simulink model "F4PhantomRunningModel2021a"  (R2021a)
settings: Solver=ode4  StartTime=0.0  StopTime=tf  FixedStep=Ts  RelTol=1e-3
model workspace (MAT data in the model file):
  PositionStateAttributes = {'Xe', 'Ye', 'Ze'}
  QuaternionStateAttributes = {'qr', 'qi', 'qj', 'qk'}
  RotationStateAttributes = {'p', 'q', 'r'}
  VelocityStateAttributes = {'U', 'v', 'w'}
values from neighbouring files (symbols this model uses):
  Hw3Coeffs = [c_L_alpha c_L_delta_E c_L_i_H c_m_alpha c_m_delta_E c_m_i_H c_L_alphadot c_L_q c_m_alphadot c_m_q c_D_alpha]    [F4ModelCode.m]    (also in F4ModelCodeV2.m; F4ModelCodeV2Q2PartD.m; F4PhantomModelCode.m = [c_L_alpha c_L_delta_E c_L_i_H c_m_alpha c_m_delta_E c_m_i_H)
  Hw4Coeffs = [c_Y_beta c_Y_delta_A c_Y_delta_R c_n_beta c_n_delta_A c_n_delta_R c_l_beta c_l_delta_A c_l_delta_R c_l_p c_Y_p c_n_p c_l_r c_Y_r c_n_r]    [F4ModelCode.m]    (also in F4ModelCodeV2.m; F4ModelCodeV2Q2PartD.m; F4PhantomModelCode.m)
  InitialInputs = [qbar1 S_ft2 c_D_1 c_L_1 cbar_ft c_m_1 uv b_ft alphadot]    [F4ModelCode.m]    (also in F4ModelCodeV2.m; F4ModelCodeV2Q2PartD.m)
  uCoeffs = [c_L_u c_D_u c_m_u]    [F4ModelCode.m]    (also in F4ModelCodeV2.m; F4ModelCodeV2Q2PartD.m; F4PhantomModelCode.m = [c_L_u c_D_u])
  uk = [c_D_delta_E c_D_q c_D_i_H c_Y_1 c_Y_betadot c_l_betadot c_n_1 c_n_betadot]    [F4ModelCode.m]    (also in F4ModelCodeV2.m; F4ModelCodeV2Q2PartD.m)
  V_P_1 = 875.6    [F4ModelCode.m]    (also in F4ModelCodeV2.m; F4ModelCodeV2Q2PartD.m; F4PhantomModelCode.m = 0)
libraries: shared6dof x1
settings Model: Creator=Owner  LastModifiedBy=billy
settings DataIOCC: ReturnWorkspaceOutputs=off
settings HardwareCC: ProdHWDeviceType=AMD->x86-64 (Windows64)
settings RTWCC: Description=Generic Real-Time Target  DLArmComputeVersion=20.02.1

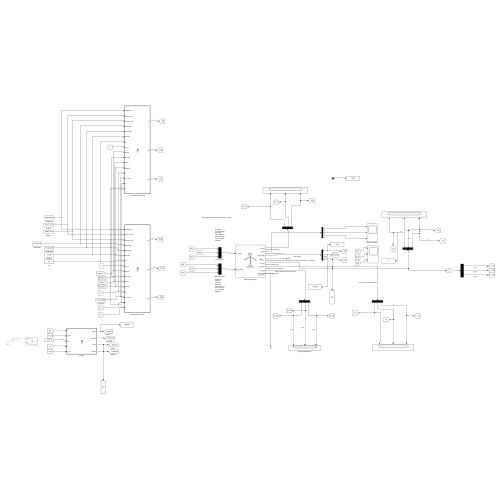
[thumbnail: Simulink's stored preview of the top-level diagram]
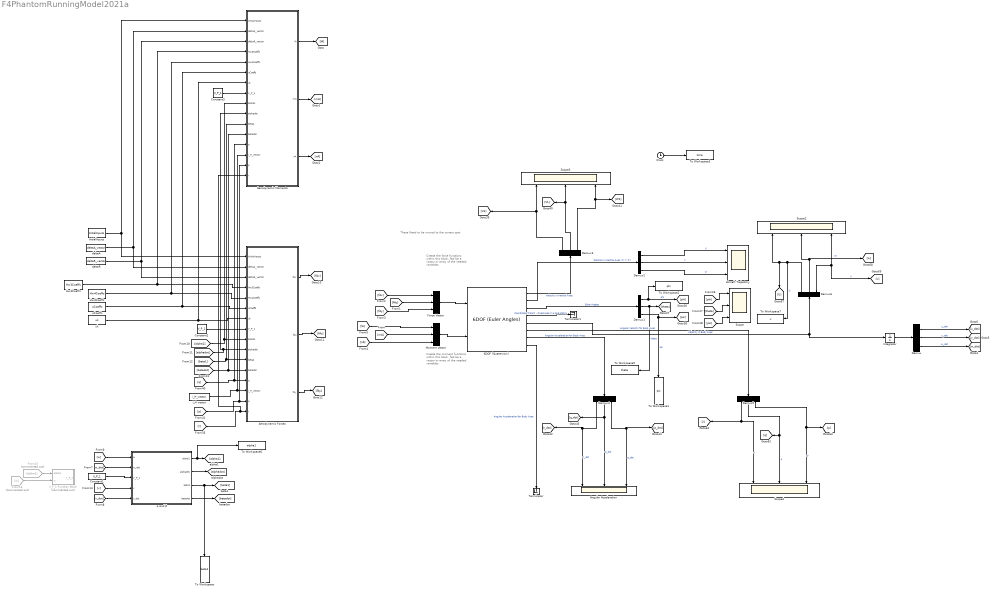
== system F4PhantomRunningModel2021a ==
  note: These Need to be moved to the correct spot
  note: Create the moment functions within this block, fed be a vector or array of the needed variables
  note: Create the force functions within this block, fed be a vector or array of the needed variables
  6DOF (Quaternion) : shared6dof/6DOF (Euler Angles)  units=English (Velocity in ft/s)  mtype=Fixed  rep=Quaternion  xme_0=InitialInertialPosition  Vm_0=InitialVelocity  eul_0=InitialEulerOrientation  pm_0=InitialRotationRates  mass_0=mass  mass_e=0.5  mass_f=2.0  inertia=I  inertia_e=eye(3)  inertia_f=2*eye(3)  k_quat=1.0  vre_flag=on  abi_flag=off  aMode=0  xme_statename=PositionStateAttributes  Vm_statename=VelocityStateAttributes  eul_statename=''  quat_statename=QuaternionStateAttributes  pm_statename=RotationStateAttributes  mass_statename=''
  Aerodynamic Forces : MATLAB Function  TreatAsAtomicUnit=on
  Aerodynamic Moments : MATLAB Function  TreatAsAtomicUnit=on
  Aircraft Trajectory : Scope  NumInputPorts=3
  Angular Acceleration : Scope  NumInputPorts=3
  Clock : Clock
  Constant1 : Constant  Value=V_P_1
  Constant2 : Constant  Value=V_P_1
  Constant3 : Constant  Value=V_P_1
  Demux{,1..6} (7 alike) : Demux  Outputs=3
  Force Vector : Mux  Inputs=3
  From15 : From  Commented=on  GotoTag=alpha1
  From16 : From  Commented=on  GotoTag=w
  Hw3Coeffs : Constant  Value=Hw3Coeffs
  Hw4Coeffs : Constant  Value=Hw4Coeffs
  InitialInputs : Constant  Value=InitialInputs
  Integrator : Integrator
  Moment Vector : Mux  Inputs=3
  Scope{,2..4} (4 alike) : Scope  NumInputPorts=3
  Terminator : Terminator
  Terminator1 : Terminator
  To Workspace : ToWorkspace  VariableName=beta1  SampleTime=-1
      settings: Save2DSignal=2-D array (concatenate along first dimension)
  To Workspace1 : ToWorkspace  VariableName=psi  SampleTime=-1
      settings: Save2DSignal=2-D array (concatenate along first dimension)
  To Workspace2 : ToWorkspace  VariableName=phi  SampleTime=-1
      settings: Save2DSignal=2-D array (concatenate along first dimension)
  To Workspace3 : ToWorkspace  VariableName=time  SaveFormat=Timeseries  SampleTime=-1
  To Workspace5 : ToWorkspace  VariableName=theta  SampleTime=-1
      settings: Save2DSignal=2-D array (concatenate along first dimension)
  To Workspace6 : ToWorkspace  VariableName=alpha1  SampleTime=-1
      settings: Save2DSignal=2-D array (concatenate along first dimension)
  To Workspace7 : ToWorkspace  VariableName=u  SampleTime=-1
      settings: Save2DSignal=2-D array (concatenate along first dimension)
  V_P_1 Function Block : MATLAB Function  Commented=on  TreatAsAtomicUnit=on
  "deltaA " : FromWorkspace  VariableName=deltaA_vector  OutDataTypeStr=double
  "deltaR " : FromWorkspace  VariableName=deltaR_vector  OutDataTypeStr=double
  "i_H vector " : FromWorkspace  VariableName=i_H_vector
  uCoeffs : Constant  Value=uCoeffs
  uk : Constant  Value=uk
  α and β : MATLAB Function  TreatAsAtomicUnit=on
  wires:
  Force Vector/1 -> 6DOF (Quaternion)/1
  6DOF (Quaternion)/1 -> Demux3/1  "Velocity in Inertial Axes"
  6DOF (Quaternion)/2 -> Demux2/1  "Position in Inertial Axes (X' Y' Z')"
  6DOF (Quaternion)/3 -> Demux1/1  "Euler Angles"
  6DOF (Quaternion)/4 -> Terminator1/1  "Coordinate Transformation from Flat Earth axes to Body-Fixed axes in a 3x3 Matrix"
  6DOF (Quaternion)/5 -> Integrator/1, Demux6/1  "Velocity in Body Axes"
  6DOF (Quaternion)/6 -> Demux5/1  "Angular Velocity for Body Axes"
  6DOF (Quaternion)/7 -> Demux4/1  "Angular Acceleration for Body Axes"
  6DOF (Quaternion)/8 -> Terminator/1  "Angular Acceleration for Body Axes"
  Aerodynamic Forces/1(fAx) -> [fAx]
  Aerodynamic Forces/2(fAz) -> [fAz]
  Aerodynamic Forces/3(fAy) -> [fAy]
  Moment Vector/1 -> 6DOF (Quaternion)/2
  [fAz] -> Force Vector/2
  [fAx] -> Force Vector/1
  [mA] -> Moment Vector/2
  [fAy] -> Force Vector/3
  [nA] -> Moment Vector/3
  [lA] -> Moment Vector/1
  Demux1/1 -> To Workspace2/1, [phi]  "phi"
  Demux1/2 -> To Workspace5/1, [theta]  "theta"
  Demux1/3 -> [psi], To Workspace1/1  "psi"
  [phi] -> Scope/1
  [theta] -> Scope/2
  [psi] -> Scope/3
  Demux2/1 -> Aircraft Trajectory/1  "X'"
  Demux2/2 -> Aircraft Trajectory/2  "Y'"
  Demux2/3 -> Aircraft Trajectory/3  "Z'"
  Demux3/1 -> Scope3/1, [U1]
  Demux3/2 -> [V1], Scope3/2
  Demux3/3 -> Scope3/3, [W1]
  Demux4/1 -> [r_dot], Angular Acceleration/1  "r_dot"
  Demux4/2 -> [q_dot], Angular Acceleration/2  "q_dot"
  Demux4/3 -> [p_dot], Angular Acceleration/3  "p_dot"
  Demux5/1 -> [r], Scope4/1  "r"
  Demux5/2 -> [q], Scope4/2  "q"
  Demux5/3 -> [p], Scope4/3  "p"
  [p] -> Aerodynamic Moments/15(p), Aerodynamic Forces/15(p)
  [r] -> Aerodynamic Moments/16(r), Aerodynamic Forces/16(r)
  α and β/1(alpha1) -> To Workspace6/1, [alpha1]
  α and β/4(betadot) -> [betadot]
  α and β/3(beta1) -> [beta1], To Workspace/1
  α and β/2(alphadot) -> [alphadot]
  Demux6/3 -> [v], Scope2/3  "V"
  Demux6/2 -> [w], Scope2/2  "W"
  Demux6/1 -> To Workspace7/1, Scope2/1, [U]  "U"
  [q] -> Aerodynamic Moments/13(q), Aerodynamic Forces/13(q)
  InitialInputs/1 -> Aerodynamic Moments/1(InitialInputs), Aerodynamic Forces/1(InitialInputs)
  "deltaA "/1 -> Aerodynamic Moments/2(deltaA_vector), Aerodynamic Forces/2(deltaA_vector)
  Hw3Coeffs/1 -> Aerodynamic Moments/4(Hw3Coeffs), Aerodynamic Forces/4(Hw3Coeffs)
  Hw4Coeffs/1 -> Aerodynamic Moments/5(Hw4Coeffs), Aerodynamic Forces/5(Hw4Coeffs)
  uCoeffs/1 -> Aerodynamic Moments/6(uCoeffs), Aerodynamic Forces/6(uCoeffs)
  uk/1 -> Aerodynamic Moments/7(uk), Aerodynamic Forces/7(uk)
  "i_H vector "/1 -> Aerodynamic Moments/14(i_H_vector), Aerodynamic Forces/14(i_H_vector)
  [alpha1] -> Aerodynamic Forces/9(alpha1), Aerodynamic Moments/9(alpha1)
  [alphadot] -> Aerodynamic Forces/10(alphadot), Aerodynamic Moments/10(alphadot)
  [beta1] -> Aerodynamic Forces/11(beta1), Aerodynamic Moments/11(beta1)
  [betadot] -> Aerodynamic Forces/12(betadot), Aerodynamic Moments/12(betadot)
  Integrator/1 -> Demux/1
  Demux/1 -> [u_dot]  "u_dot"
  Demux/2 -> [v_dot]  "v_dot"
  Demux/3 -> [w_dot]  "w_dot"
  [w_dot] -> α and β/2(w_dot)
  [v_dot] -> α and β/5(v_dot)
  [w] -> α and β/1(w)
  [v] -> α and β/4(v)
  From15/1 -> V_P_1 Function Block/1(alpha1)
  From16/1 -> V_P_1 Function Block/2(w)
  "deltaR "/1 -> Aerodynamic Moments/3(deltaR_vector), Aerodynamic Forces/3(deltaR_vector)
  Aerodynamic Moments/1(lA) -> [lA]
  Aerodynamic Moments/2(mA) -> [mA]
  Aerodynamic Moments/3(nA) -> [nA]
  Constant1/1 -> α and β/3(V_P_1)
  Constant2/1 -> Aerodynamic Forces/8(V_P_1)
  Constant3/1 -> Aerodynamic Moments/8(V_P_1)
  Clock/1 -> To Workspace3/1

== matlab function F4PhantomRunningModel2021a/Aerodynamic Forces ==
  data: InitialInputs input; deltaA_vector input; deltaR_vector input; Hw3Coeffs input; Hw4Coeffs input; uCoeffs input; uk input; V_P_1 input; alpha1 input; alphadot input; beta1 input; betadot input; q input; i_H_vector input; fAx output; fAz output; fAy output; p input; r input
function [ fAx, fAz,  fAy]  = fcn(InitialInputs, deltaA_vector, deltaR_vector, Hw3Coeffs, Hw4Coeffs, uCoeffs, uk, V_P_1, alpha1, alphadot, beta1, betadot, q, i_H_vector, p, r)
qbar1 = InitialInputs(1); S_ft2 = InitialInputs(2); c_D_1 = InitialInputs(3); c_L_1 = InitialInputs(4); cbar_ft = InitialInputs(5); c_m_1 = InitialInputs(6); uv = InitialInputs(7); b_ft = InitialInputs(8);
% deltaA_vector = CSv(1); deltaR_vector = CSv(2); deltaS_vector = CSv(3); 
% deltaA = CSc(1); deltaS = CSc(2); deltaR = CSc(3);
c_L_alpha = Hw3Coeffs(1); c_L_delta_E = Hw3Coeffs(2); c_L_i_H = Hw3Coeffs(3); c_m_alpha = Hw3Coeffs(4); c_m_delta_E = Hw3Coeffs(5); c_m_i_H = Hw3Coeffs(6); c_L_alphadot = Hw3Coeffs(7); c_L_q = Hw3Coeffs(8); c_m_alphadot = Hw3Coeffs(9); c_m_q = Hw3Coeffs(10); c_D_alpha = Hw3Coeffs(11);
c_Y_beta = Hw4Coeffs(1); c_Y_delta_A = Hw4Coeffs(2); c_Y_delta_R = Hw4Coeffs(3); c_n_beta = Hw4Coeffs(4); c_n_delta_A = Hw4Coeffs(5); c_n_delta_R = Hw4Coeffs(6); c_l_beta = Hw4Coeffs(7); c_l_delta_A = Hw4Coeffs(8); c_l_delta_R = Hw4Coeffs(9); c_l_p = Hw4Coeffs(10); c_Y_p = Hw4Coeffs(11); c_n_p = Hw4Coeffs(12); c_l_r = Hw4Coeffs(13); c_Y_r = Hw4Coeffs(14); c_n_r = Hw4Coeffs(15);
c_L_u = uCoeffs(1); c_D_u = uCoeffs(2); c_m_u = uCoeffs(3); 
c_D_delta_E = uk(1);  c_D_q = uk(2); c_D_i_H = uk(3); c_Y_1 = uk(4); c_Y_betadot = uk(5); c_l_betadot = uk(6); c_n_1 = uk(7); c_n_betadot = uk(8);

deltaE = 0;

%FAx = -qbar1*S_ft2*c_D_1;
fAx = (qbar1*S_ft2)*(((-(c_D_u+(2*c_D_1)))*(uv/V_P_1)) + ((c_D_alpha + c_L_1)*(alpha1)) - c_D_alpha*((alphadot*cbar_ft)/(2*V_P_1)) - c_D_q*((q*cbar_ft)/(2*V_P_1)) - (c_D_delta_E*deltaE)-(c_D_i_H*i_H_vector));

%FAz = -qbar1*S_ft2*c_L_1;
fAz = (qbar1*S_ft2)*(((-(c_L_u+(2*c_L_1)))*(uv/V_P_1)) + ((c_L_alpha + c_D_1)*(alpha1)) - c_L_alphadot*((alphadot*cbar_ft)/(2*V_P_1)) - c_L_q*((q*cbar_ft)/(2*V_P_1)) - (c_L_delta_E*deltaE)-(c_L_i_H*i_H_vector));

%FAy = -qbar1*S_ft2*c_Y_1;
fAy = -qbar1*S_ft2 * ((c_Y_beta*beta1) + c_Y_betadot * ((betadot*b_ft)/(2*V_P_1)) + c_Y_p*((p*b_ft)/(2*V_P_1)) + c_Y_r * ((r*b_ft)/(2*V_P_1)) +(c_Y_delta_A * deltaA_vector) + (c_Y_delta_R*deltaR_vector));

%LA = -qbar1*S_ft2*b_ft*c_L_1;
% lA = -qbar1*S_ft2*b_ft*((c_l_beta*beta1) + c_l_betadot * ((betadot*b_ft)/(2*V_P_1)) + c_l_p*((p*b_ft)/(2*V_P_1)) + c_l_r * ((r*b_ft)/(2*V_P_1)) +(c_l_delta_A * deltaA_vector) + (c_l_delta_R*deltaR_vector));
% 
% %MA = -qbar1*S_ft2*cbar_ft*c_m_1; %%%%This line is throwing an error
% mA = (qbar1*S_ft2*cbar_ft)*(((-(c_m_u+(2*c_m_1)))*(uv/V_P_1)) + (c_m_alpha*alpha1) + c_m_alphadot*((alphadot*cbar_ft)/(2*V_P_1)) + c_m_q*((q*cbar_ft)/(2*V_P_1)) + (c_m_delta_E*deltaE)+(c_L_i_H*i_H_vector));
% 
% %NA = -qbar1*S_ft2*b_ft*c_n_1;
% nA = -qbar1*S_ft2*b_ft*((c_n_beta*beta1) + c_n_betadot * ((betadot*b_ft)/(2*V_P_1)) + c_n_p*((p*b_ft)/(2*V_P_1)) + c_n_r * ((r*b_ft)/(2*V_P_1)) +(c_n_delta_A * deltaA_vector) + (c_n_delta_R*deltaR_vector));

%Need to get rid of fAy and lA and nA, leave MA and mA

== matlab function F4PhantomRunningModel2021a/α and β ==
  data: w input; alpha1 output; alphadot output; beta1 output; w_dot input; V_P_1 input; v input; v_dot input; betadot output
function [alpha1, alphadot, beta1, betadot] = fcn(w, w_dot, V_P_1, v, v_dot)

alpha1 = w/V_P_1;

alphadot = w_dot/V_P_1;

beta1 = v/V_P_1;

betadot = v_dot/V_P_1;

== matlab function F4PhantomRunningModel2021a/V_P_1 Function Block ==
  data: alpha1 input; V_P_1 output; w input
function V_P_1 = fcn(alpha1,w)

alpha1 = deg2rad(alpha1); 
V_P_1 = w/alpha1;

== matlab function F4PhantomRunningModel2021a/Aerodynamic Moments ==
  data: InitialInputs input; deltaA_vector input; deltaR_vector input; Hw3Coeffs input; Hw4Coeffs input; uCoeffs input; uk input; V_P_1 input; alpha1 input; alphadot input; beta1 input; betadot input; q input; i_H_vector input; lA output; mA output; nA output; p input; r input
function [lA,  mA, nA]  = fcn(InitialInputs, deltaA_vector, deltaR_vector, Hw3Coeffs, Hw4Coeffs, uCoeffs, uk, V_P_1, alpha1, alphadot, beta1, betadot, q, i_H_vector, p, r)
qbar1 = InitialInputs(1); S_ft2 = InitialInputs(2); c_D_1 = InitialInputs(3); c_L_1 = InitialInputs(4); cbar_ft = InitialInputs(5); c_m_1 = InitialInputs(6); uv = InitialInputs(7); b_ft = InitialInputs(8);
% deltaA_vector = CSv(1); deltaR_vector = CSv(2); deltaS_vector = CSv(3); 
% deltaA = CSc(1); deltaS = CSc(2); deltaR = CSc(3);
c_L_alpha = Hw3Coeffs(1); c_L_delta_E = Hw3Coeffs(2); c_L_i_H = Hw3Coeffs(3); c_m_alpha = Hw3Coeffs(4); c_m_delta_E = Hw3Coeffs(5); c_m_i_H = Hw3Coeffs(6); c_L_alphadot = Hw3Coeffs(7); c_L_q = Hw3Coeffs(8); c_m_alphadot = Hw3Coeffs(9); c_m_q = Hw3Coeffs(10); c_D_alpha = Hw3Coeffs(11);
c_Y_beta = Hw4Coeffs(1); c_Y_delta_A = Hw4Coeffs(2); c_Y_delta_R = Hw4Coeffs(3); c_n_beta = Hw4Coeffs(4); c_n_delta_A = Hw4Coeffs(5); c_n_delta_R = Hw4Coeffs(6); c_l_beta = Hw4Coeffs(7); c_l_delta_A = Hw4Coeffs(8); c_l_delta_R = Hw4Coeffs(9); c_l_p = Hw4Coeffs(10); c_Y_p = Hw4Coeffs(11); c_n_p = Hw4Coeffs(12); c_l_r = Hw4Coeffs(13); c_Y_r = Hw4Coeffs(14); c_n_r = Hw4Coeffs(15);
c_L_u = uCoeffs(1); c_D_u = uCoeffs(2); c_m_u = uCoeffs(3); 
c_D_delta_E = uk(1);  c_D_q = uk(2); c_D_i_H = uk(3); c_Y_1 = uk(4); c_Y_betadot = uk(5); c_l_betadot = uk(6); c_n_1 = uk(7); c_n_betadot = uk(8);

deltaE = 0;

% %FAx = -qbar1*S_ft2*c_D_1;
% fAx = (qbar1*S_ft2)*(((-(c_D_u+(2*c_D_1)))*(uv/V_P_1)) + ((c_D_alpha + c_L_1)*(alpha1)) - c_D_alpha*((alphadot*cbar_ft)/(2*V_P_1)) - c_D_q*((q*cbar_ft)/(2*V_P_1)) - (c_D_delta_E*deltaE)-(c_D_i_H*i_H_vector));
% 
% %FAz = -qbar1*S_ft2*c_L_1;
% fAz = (qbar1*S_ft2)*(((-(c_L_u+(2*c_L_1)))*(uv/V_P_1)) + ((c_L_alpha + c_D_1)*(alpha1)) - c_L_alphadot*((alphadot*cbar_ft)/(2*V_P_1)) - c_L_q*((q*cbar_ft)/(2*V_P_1)) - (c_L_delta_E*deltaE)-(c_L_i_H*i_H_vector));
% 
% %FAy = -qbar1*S_ft2*c_Y_1;
% fAy = -qbar1*S_ft2 * ((c_Y_beta*beta1) + c_Y_betadot * ((betadot*b_ft)/(2*V_P_1)) + c_Y_p*((p*b_ft)/(2*V_P_1)) + c_Y_r * ((r*b_ft)/(2*V_P_1)) +(c_Y_delta_A * deltaA_vector) + (c_Y_delta_R*deltaR_vector));

%LA = -qbar1*S_ft2*b_ft*c_L_1;
lA = -qbar1*S_ft2*b_ft*((c_l_beta*beta1) + c_l_betadot * ((betadot*b_ft)/(2*V_P_1)) + c_l_p*((p*b_ft)/(2*V_P_1)) + c_l_r * ((r*b_ft)/(2*V_P_1)) +(c_l_delta_A * deltaA_vector) + (c_l_delta_R*deltaR_vector));
% 
% %MA = -qbar1*S_ft2*cbar_ft*c_m_1; %%%%This line is throwing an error
mA = (qbar1*S_ft2*cbar_ft)*(((-(c_m_u+(2*c_m_1)))*(uv/V_P_1)) + (c_m_alpha*alpha1) + c_m_alphadot*((alphadot*cbar_ft)/(2*V_P_1)) + c_m_q*((q*cbar_ft)/(2*V_P_1)) + (c_m_delta_E*deltaE)+(c_L_i_H*i_H_vector));
% 
% %NA = -qbar1*S_ft2*b_ft*c_n_1;
nA = -qbar1*S_ft2*b_ft*((c_n_beta*beta1) + c_n_betadot * ((betadot*b_ft)/(2*V_P_1)) + c_n_p*((p*b_ft)/(2*V_P_1)) + c_n_r * ((r*b_ft)/(2*V_P_1)) +(c_n_delta_A * deltaA_vector) + (c_n_delta_R*deltaR_vector));

%Need to get rid of fAy and lA and nA, leave MA and mA
